simulink model "RangeSensorState1"  (R2017b)
settings: Solver=VariableStepAuto  StartTime=0.0  StopTime=10.0  RelTol=1e-3
libraries: realtime_pacer_lib x1
settings Model: Creator=wafflefries  LastModifiedBy=wafflefries

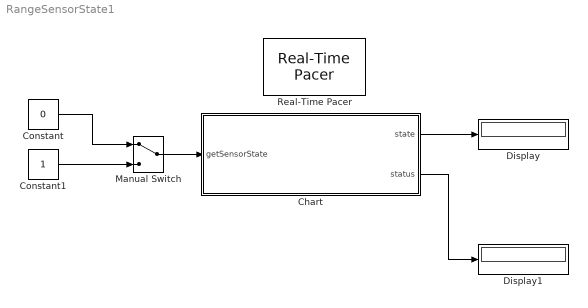
== system RangeSensorState1 ==
  Chart : Stateflow chart  TreatAsAtomicUnit=on
  Constant : Constant  Value=0
  Constant1 : Constant
  Display : Display
  Display1 : Display
  Manual Switch : ManualSwitch
  Real-Time Pacer : realtime_pacer_lib/Real-Time Pacer  simTimePerRealTime=0.5
  wires:
  Manual Switch/1 -> Chart/1(getSensorState)
  Constant/1 -> Manual Switch/1
  Constant1/1 -> Manual Switch/2
  Chart/1(state) -> Display/1
  Chart/2(status) -> Display1/1

== stateflow chart RangeSensorState1/Chart ==
  state NOOP
    entry:
    status = 0;
  state START
    entry:
    coder.extrinsic('RangeStateRoomba')
    state = RangeStateRoomba(so)
    status = 1;
  state RESET
    entry:
  (default) -> NOOP : {
      | coder.extrinsic('RoombaWiFiInit')
      | so = RoombaWiFiInit(' ', 'full')
      | }
  RESET -> NOOP
  NOOP -> START : [getSensorState == 1]
  START -> RESET : [getSensorState == 0]
  data: state output size=6; getSensorState input; status output; so local
